simulink model "ADMIRE"  (R2021b)
settings: Solver=ode4  StartTime=0.0  StopTime=100  FixedStep=1e-2  RelTol=1e-3
undefined symbols (not defined in the file or in its folder): admireDB, Earth, WGS84
libraries: simulink_extras x112, simulink x27, aerolibutil x4, dspsigops x4, aerolibfltsims x3, sharedtransform x2, aerolibtransform2 x2, aerolibatmos2 x1, matrix_library x1, sharedutil x1, aerolibanimutils x1, vrlib x1
(part 8 of 15)

== system ADMIRE/Aircraft/Aerodynamics/TangentialForceCoefficient/MachRegion3/Ctlg ==
  in_bus : Inport
  Abs : Abs
  Bus Selector : BusSelector  OutputSignals=AeroIn_Bus.angleOfAttack_deg,AeroIn_Bus.angleOfSideslip_deg,AeroIn_Bus.lg_bool
  CTLST_BETA_ALFA : Lookup_n-D  BreakpointsForDimension1=admireDB.aerodata_sym.CTLST.breakpoints.ALFA  BreakpointsForDimension2=admireDB.aerodata_sym.CTLST.breakpoints.BETA  BreakpointsForDimension3=[5, 7]  Table=admireDB.aerodata_sym.CTLST.newTable  ExtrapMethod=Clip  InternalRulePriority=Speed  RndMeth=Simplest  InputSameDT=on
      settings: InputPortMap=u0,u1
  Product : Product  Inputs=**
  Ctlg : Outport
  wires:
  Abs/1 -> CTLST_BETA_ALFA/2
  Bus Selector/3 -> Product/2  "<lg_bool>"
  CTLST_BETA_ALFA/1 -> Product/1
  in_bus/1 -> Bus Selector/1
  Bus Selector/2 -> Abs/1  "<angleOfSideslip_deg>"
  Bus Selector/1 -> CTLST_BETA_ALFA/1  "<angleOfAttack_deg>"
  Product/1 -> Ctlg/1

== system ADMIRE/Aircraft/Aerodynamics/TangentialForceCoefficient/MachRegion3/eoeff ==
  AeroIn_Bus : Inport
  Bus Selector : BusSelector  OutputSignals=mach_nd
  CTDEYODE_M : Lookup_n-D  NumberOfTableDimensions=1  BreakpointsForDimension1=admireDB.aerodata_sym.CTDEYODE.breakpoints.M  BreakpointsForDimension3=[5, 7]  Table=admireDB.aerodata_sym.CTDEYODE.newTable  ExtrapMethod=Clip  InternalRulePriority=Speed  RndMeth=Simplest  InputSameDT=on
  Constant : Constant
  Sum : Sum  Inputs=-+|
  eoeff : Outport
  eieff : Outport  Port=2
  wires:
  Sum/1 -> eieff/1
  CTDEYODE_M/1 -> eoeff/1, Sum/1
  Constant/1 -> Sum/2
  Bus Selector/1 -> CTDEYODE_M/1  "<mach_nd>"
  AeroIn_Bus/1 -> Bus Selector/1

== system ADMIRE/Aircraft/Aerodynamics/YawMomentCoefficient/MachRegion1/Cymbasic ==
  in_bus : Inport
  Bus Selector : BusSelector  OutputSignals=AeroIn_Bus.angleOfAttack_deg
  Cymbasic_ : Subsystem
  Cymbasic : Outport
  wires:
  Cymbasic_/1(Cymbasic) -> Cymbasic/1
  Bus Selector/1 -> Cymbasic_/1(angleOfAttack_deg)  "<angleOfAttack_deg>"
  in_bus/1 -> Bus Selector/1  "in_bus"

== system ADMIRE/Aircraft/Aerodynamics/YawMomentCoefficient/MachRegion1/Cymbcai ==
  in_bus : Inport
  Bus Selector : BusSelector  OutputSignals=AeroIn_Bus.cai,AeroIn_Bus.angleOfAttack_deg,AeroIn_Bus.angleOfSideslip_deg
  Cymbcai_ : Subsystem
  Cymbcai : Outport
  wires:
  Bus Selector/3 -> Cymbcai_/3(angleOfSideslip_deg)  "<angleOfSideslip_deg>"
  Bus Selector/2 -> Cymbcai_/2(angleOfAttack_deg)  "<angleOfAttack_deg>"
  Bus Selector/1 -> Cymbcai_/1(CAI)  "<cai>"
  in_bus/1 -> Bus Selector/1  "in_bus"
  Cymbcai_/1(Cymbcai) -> Cymbcai/1

== system ADMIRE/Aircraft/Aerodynamics/YawMomentCoefficient/MachRegion1/Cymbde ==
  in_bus : Inport
  Bus Selector : BusSelector  OutputSignals=AeroIn_Bus.angleOfAttack_deg,AeroIn_Bus.dEI,AeroIn_Bus.angleOfSideslip_deg,AeroIn_Bus.dEY,eieff,eoeff
  Cymbde_ : Subsystem
  Cymbde : Outport
  wires:
  Bus Selector/6 -> Cymbde_/6(eoeff)  "<eoeff>"
  Bus Selector/5 -> Cymbde_/5(eieff)  "<eieff>"
  Bus Selector/4 -> Cymbde_/4(dEY)  "<dEY>"
  Bus Selector/3 -> Cymbde_/3(angleOfSideslip_deg)  "<angleOfSideslip_deg>"
  Bus Selector/2 -> Cymbde_/2(dEI)  "<dEI>"
  Bus Selector/1 -> Cymbde_/1(angleOfAttack_deg)  "<angleOfAttack_deg>"
  Cymbde_/1(Cymbde) -> Cymbde/1
  in_bus/1 -> Bus Selector/1  "in_bus"

== system ADMIRE/Aircraft/Aerodynamics/YawMomentCoefficient/MachRegion1/Cymbdle ==
  in_bus : Inport
  Bus Selector : BusSelector  OutputSignals=AeroIn_Bus.angleOfAttack_deg,AeroIn_Bus.dEI,AeroIn_Bus.angleOfSideslip_deg,AeroIn_Bus.lef_deg,AeroIn_Bus.dEY,eieff,eoeff
  Cymbdle_ : Subsystem
  Cymbdle : Outport
  wires:
  Bus Selector/2 -> Cymbdle_/2(dEI)  "<dEI>"
  Bus Selector/1 -> Cymbdle_/1(angleOfAttack_deg)  "<angleOfAttack_deg>"
  Bus Selector/3 -> Cymbdle_/3(angleOfSideslip_deg)  "<angleOfSideslip_deg>"
  Bus Selector/4 -> Cymbdle_/4(dLE)  "<lef_deg>"
  Bus Selector/5 -> Cymbdle_/5(dEY)  "<dEY>"
  Bus Selector/6 -> Cymbdle_/6(eieff)  "<eieff>"
  Bus Selector/7 -> Cymbdle_/7(eoeff)  "<eoeff>"
  Cymbdle_/1(Cymbdle) -> Cymbdle/1
  in_bus/1 -> Bus Selector/1  "in_bus"

== system ADMIRE/Aircraft/Aerodynamics/YawMomentCoefficient/MachRegion1/Cymbdn ==
  in_bus : Inport
  Bus Selector : BusSelector  OutputSignals=AeroIn_Bus.angleOfAttack_deg,AeroIn_Bus.dN,AeroIn_Bus.angleOfSideslip_deg
  Cymbdn_ : Subsystem
  Cymbdn : Outport
  wires:
  Bus Selector/1 -> Cymbdn_/1(angleOfAttack_deg)  "<angleOfAttack_deg>"
  Bus Selector/3 -> Cymbdn_/3(angleOfSideslip_deg)  "<angleOfSideslip_deg>"
  Bus Selector/2 -> Cymbdn_/2(dN)  "<dN>"
  in_bus/1 -> Bus Selector/1  "in_bus"
  Cymbdn_/1(Cymbdn) -> Cymbdn/1

== system ADMIRE/Aircraft/Aerodynamics/YawMomentCoefficient/MachRegion1/Cymbeta ==
  in_bus : Inport
  Bus Selector : BusSelector  OutputSignals=AeroIn_Bus.angleOfSideslip_deg,AeroIn_Bus.angleOfAttack_deg,AeroIn_Bus.qacorr,AeroIn_Bus.mach_nd
  Cymbeta_ : Subsystem
  Cymbeta : Outport
  wires:
  Bus Selector/4 -> Cymbeta_/4(mach_nd)  "<mach_nd>"
  Bus Selector/3 -> Cymbeta_/3(qacorr)  "<qacorr>"
  Bus Selector/2 -> Cymbeta_/2(angleOfAttack_deg)  "<angleOfAttack_deg>"
  Bus Selector/1 -> Cymbeta_/1(angleOfSideslip_deg)  "<angleOfSideslip_deg>"
  in_bus/1 -> Bus Selector/1  "in_bus"
  Cymbeta_/1(Cymbeta) -> Cymbeta/1

== system ADMIRE/Aircraft/Aerodynamics/YawMomentCoefficient/MachRegion1/Cymbetad ==
  in_bus : Inport
  Bus Selector : BusSelector  OutputSignals=AeroIn_Bus.angleOfAttack_deg,AeroIn_Bus.betad
  Cymbetad_ : Subsystem
  Cymbetad : Outport
  wires:
  Bus Selector/1 -> Cymbetad_/1(angleOfAttack_deg)  "<angleOfAttack_deg>"
  Bus Selector/2 -> Cymbetad_/2(betad)  "<betad>"
  Cymbetad_/1(Cymbetad) -> Cymbetad/1
  in_bus/1 -> Bus Selector/1  "in_bus"

== system ADMIRE/Aircraft/Aerodynamics/YawMomentCoefficient/MachRegion1/Cymblg ==
  in_bus : Inport
  Bus Selector : BusSelector  OutputSignals=AeroIn_Bus.angleOfSideslip_deg,AeroIn_Bus.lg_bool,AeroIn_Bus.angleOfAttack_deg
  Cymblg_ : Subsystem
  Cymblg : Outport
  wires:
  Bus Selector/3 -> Cymblg_/3(angleOfAttack_deg)  "<angleOfAttack_deg>"
  Bus Selector/1 -> Cymblg_/1(angleOfSideslip_deg)  "<angleOfSideslip_deg>"
  Bus Selector/2 -> Cymblg_/2(dLG)  "<lg_bool>"
  Cymblg_/1(Cymblg) -> Cymblg/1
  in_bus/1 -> Bus Selector/1  "in_bus"

== system ADMIRE/Aircraft/Aerodynamics/YawMomentCoefficient/MachRegion1/Cymdai ==
  in_bus : Inport
  Bus Selector : BusSelector  OutputSignals=AeroIn_Bus.dAI,AeroIn_Bus.angleOfAttack_deg,AeroIn_Bus.dEI,eieff,AeroIn_Bus.qacorr,AeroIn_Bus.mach_nd
  Cymdai_ : Subsystem
  Cymdai : Outport
  wires:
  Bus Selector/1 -> Cymdai_/1(dAI)  "<dAI>"
  Bus Selector/2 -> Cymdai_/2(angleOfAttack_deg)  "<angleOfAttack_deg>"
  Bus Selector/3 -> Cymdai_/3(dEI)  "<dEI>"
  Bus Selector/4 -> Cymdai_/4(eieff)  "<eieff>"
  Bus Selector/5 -> Cymdai_/5(qacorr)  "<qacorr>"
  Bus Selector/6 -> Cymdai_/6(mach_nd)  "<mach_nd>"
  Cymdai_/1(Cymdai) -> Cymdai/1
  in_bus/1 -> Bus Selector/1  "in_bus"

== system ADMIRE/Aircraft/Aerodynamics/YawMomentCoefficient/MachRegion1/Cymdaib ==
  in_bus : Inport
  Bus Selector : BusSelector  OutputSignals=AeroIn_Bus.angleOfAttack_deg,AeroIn_Bus.dAI,AeroIn_Bus.angleOfSideslip_deg,eieff
  Cymdaib_ : Subsystem
  Cymdaib : Outport
  wires:
  Bus Selector/4 -> Cymdaib_/4(eieff)  "<eieff>"
  Bus Selector/3 -> Cymdaib_/3(angleOfSideslip_deg)  "<angleOfSideslip_deg>"
  Bus Selector/2 -> Cymdaib_/2(dAI)  "<dAI>"
  Bus Selector/1 -> Cymdaib_/1(angleOfAttack_deg)  "<angleOfAttack_deg>"
  Cymdaib_/1(Cymdaib) -> Cymdaib/1
  in_bus/1 -> Bus Selector/1  "in_bus"

== system ADMIRE/Aircraft/Aerodynamics/YawMomentCoefficient/MachRegion1/Cymday ==
  in_bus : Inport
  Bus Selector : BusSelector  OutputSignals=AeroIn_Bus.dAY,AeroIn_Bus.angleOfAttack_deg,AeroIn_Bus.dEY,eoeff,AeroIn_Bus.qacorr,AeroIn_Bus.mach_nd
  Cymday_ : Subsystem
  Cymday : Outport
  wires:
  Bus Selector/1 -> Cymday_/1(dAY)  "<dAY>"
  Bus Selector/2 -> Cymday_/2(angleOfAttack_deg)  "<angleOfAttack_deg>"
  Bus Selector/3 -> Cymday_/3(dEY)  "<dEY>"
  Bus Selector/4 -> Cymday_/4(eoeff)  "<eoeff>"
  Bus Selector/5 -> Cymday_/5(qacorr)  "<qacorr>"
  Bus Selector/6 -> Cymday_/6(mach_nd)  "<mach_nd>"
  in_bus/1 -> Bus Selector/1  "in_bus"
  Cymday_/1(Cymday) -> Cymday/1

== system ADMIRE/Aircraft/Aerodynamics/YawMomentCoefficient/MachRegion1/Cymdayb ==
  in_bus : Inport
  Bus Selector : BusSelector  OutputSignals=AeroIn_Bus.angleOfAttack_deg,AeroIn_Bus.dAY,AeroIn_Bus.angleOfSideslip_deg,eoeff
  Cymdayb_ : Subsystem
  Cymdayb : Outport
  wires:
  Bus Selector/4 -> Cymdayb_/4(eoeff)  "<eoeff>"
  Bus Selector/3 -> Cymdayb_/3(angleOfSideslip_deg)  "<angleOfSideslip_deg>"
  Bus Selector/2 -> Cymdayb_/2(dAY)  "<dAY>"
  Bus Selector/1 -> Cymdayb_/1(angleOfAttack_deg)  "<angleOfAttack_deg>"
  Cymdayb_/1(Cymdaib) -> Cymdayb/1
  in_bus/1 -> Bus Selector/1  "in_bus"

== system ADMIRE/Aircraft/Aerodynamics/YawMomentCoefficient/MachRegion1/Cymdna ==
  in_bus : Inport
  Bus Selector : BusSelector  OutputSignals=AeroIn_Bus.dNE,AeroIn_Bus.angleOfAttack_deg,AeroIn_Bus.dNA
  Cymdna_ : Subsystem
  Cymdna : Outport
  wires:
  Bus Selector/3 -> Cymdna_/3(dNA)  "<dNA>"
  Bus Selector/2 -> Cymdna_/2(angleOfAttack_deg)  "<angleOfAttack_deg>"
  Bus Selector/1 -> Cymdna_/1(dNE)  "<dNE>"
  in_bus/1 -> Bus Selector/1  "in_bus"
  Cymdna_/1(Cymdna) -> Cymdna/1

== system ADMIRE/Aircraft/Aerodynamics/YawMomentCoefficient/MachRegion1/Cymdr ==
  in_bus : Inport
  Bus Selector : BusSelector  OutputSignals=AeroIn_Bus.angleOfAttack_deg,AeroIn_Bus.rud_deg,AeroIn_Bus.angleOfSideslip_deg,AeroIn_Bus.qacorr,AeroIn_Bus.mach_nd
  Cymdr_ : Subsystem
  Cymdr : Outport
  wires:
  Bus Selector/5 -> Cymdr_/5(mach_nd)  "<mach_nd>"
  Bus Selector/4 -> Cymdr_/4(qacorr)  "<qacorr>"
  Bus Selector/3 -> Cymdr_/3(angleOfSideslip_deg)  "<angleOfSideslip_deg>"
  Bus Selector/2 -> Cymdr_/2(dR)  "<rud_deg>"
  Bus Selector/1 -> Cymdr_/1(angleOfAttack_deg)  "<angleOfAttack_deg>"
  in_bus/1 -> Bus Selector/1  "in_bus"
  Cymdr_/1(Cymdr) -> Cymdr/1

== system ADMIRE/Aircraft/Aerodynamics/YawMomentCoefficient/MachRegion1/Cymp ==
  in_bus : Inport
  Bus Selector : BusSelector  OutputSignals=AeroIn_Bus.dN,AeroIn_Bus.angleOfAttack_deg,AeroIn_Bus.qacorr,AeroIn_Bus.mach_nd,AeroIn_Bus.pc
  Cymp_ : Subsystem
  Cymp : Outport
  wires:
  Bus Selector/5 -> Cymp_/5(pc)  "<pc>"
  Bus Selector/4 -> Cymp_/4(mach_nd)  "<mach_nd>"
  Bus Selector/3 -> Cymp_/3(qacorr)  "<qacorr>"
  Bus Selector/2 -> Cymp_/2(angleOfAttack_deg)  "<angleOfAttack_deg>"
  Bus Selector/1 -> Cymp_/1(dN)  "<dN>"
  in_bus/1 -> Bus Selector/1  "in_bus"
  Cymp_/1(Cymp) -> Cymp/1

== system ADMIRE/Aircraft/Aerodynamics/YawMomentCoefficient/MachRegion1/Cympbeta ==
  in_bus : Inport
  Bus Selector : BusSelector  OutputSignals=AeroIn_Bus.angleOfSideslip_deg,AeroIn_Bus.angleOfAttack_deg,AeroIn_Bus.pc
  Cympbeta_ : Subsystem
  Cympbeta : Outport
  wires:
  Bus Selector/3 -> Cympbeta_/3(pc)  "<pc>"
  Bus Selector/2 -> Cympbeta_/2(angleOfAttack_deg)  "<angleOfAttack_deg>"
  Bus Selector/1 -> Cympbeta_/1(angleOfSideslip_deg)  "<angleOfSideslip_deg>"
  Cympbeta_/1(Cympbeta) -> Cympbeta/1
  in_bus/1 -> Bus Selector/1  "in_bus"

== system ADMIRE/Aircraft/Aerodynamics/YawMomentCoefficient/MachRegion1/Cymr ==
  in_bus : Inport
  Bus Selector : BusSelector  OutputSignals=AeroIn_Bus.dN,AeroIn_Bus.angleOfAttack_deg,AeroIn_Bus.rc,AeroIn_Bus.mach_nd,AeroIn_Bus.qacorr
  Cymr_ : Subsystem
  Cymr : Outport
  wires:
  Bus Selector/5 -> Cymr_/5(qacorr)  "<qacorr>"
  Bus Selector/4 -> Cymr_/4(mach_nd)  "<mach_nd>"
  Bus Selector/3 -> Cymr_/3(rc)  "<rc>"
  Bus Selector/2 -> Cymr_/2(angleOfAttack_deg)  "<angleOfAttack_deg>"
  Bus Selector/1 -> Cymr_/1(dN)  "<dN>"
  in_bus/1 -> Bus Selector/1  "in_bus"
  Cymr_/1(Cymr) -> Cymr/1

== system ADMIRE/Aircraft/Aerodynamics/YawMomentCoefficient/MachRegion1/Cymrbeta ==
  in_bus : Inport
  Bus Selector : BusSelector  OutputSignals=AeroIn_Bus.angleOfSideslip_deg,AeroIn_Bus.angleOfAttack_deg,AeroIn_Bus.rc
  Cymrbeta_ : Subsystem
  Cymrbeta : Outport
  wires:
  Bus Selector/3 -> Cymrbeta_/3(rc)  "<rc>"
  Bus Selector/2 -> Cymrbeta_/2(angleOfAttack_deg)  "<angleOfAttack_deg>"
  Bus Selector/1 -> Cymrbeta_/1(angleOfSideslip_deg)  "<angleOfSideslip_deg>"
  Cymrbeta_/1(Cymrbeta) -> Cymrbeta/1
  in_bus/1 -> Bus Selector/1  "in_bus"

== system ADMIRE/Aircraft/Aerodynamics/YawMomentCoefficient/MachRegion1/eoeff ==
  AeroIn_Bus : Inport
  Bus Selector : BusSelector  OutputSignals=mach_nd
  CYMDAYOD_M : Lookup_n-D  NumberOfTableDimensions=1  BreakpointsForDimension1=admireDB.aerodata_asym_ext.CYMDAYOD.breakpoints.M  BreakpointsForDimension3=[5, 7]  Table=admireDB.aerodata_asym_ext.CYMDAYOD.newTable  ExtrapMethod=Clip  InternalRulePriority=Speed  RndMeth=Simplest  InputSameDT=on
  Constant : Constant
  Sum : Sum  Inputs=-+|
  eoeff : Outport
  eieff : Outport  Port=2
  wires:
  Sum/1 -> eieff/1
  CYMDAYOD_M/1 -> eoeff/1, Sum/1
  Constant/1 -> Sum/2
  Bus Selector/1 -> CYMDAYOD_M/1  "<mach_nd>"
  AeroIn_Bus/1 -> Bus Selector/1

== system ADMIRE/Aircraft/Aerodynamics/YawMomentCoefficient/MachRegion2/Cymbasic ==
  in_bus : Inport
  Bus Selector : BusSelector  OutputSignals=AeroIn_Bus.angleOfAttack_deg,AeroIn_Bus.tflow
  Cymbasic_ : Subsystem
  Cymbasic : Outport
  wires:
  Bus Selector/2 -> Cymbasic_/2(tflow)  "<tflow>"
  Cymbasic_/1(Cymbasic) -> Cymbasic/1
  Bus Selector/1 -> Cymbasic_/1(angleOfAttack_deg)  "<angleOfAttack_deg>"
  in_bus/1 -> Bus Selector/1  "in_bus"

== system ADMIRE/Aircraft/Aerodynamics/YawMomentCoefficient/MachRegion2/Cymbcai ==
  in_bus : Inport
  Bus Selector : BusSelector  OutputSignals=AeroIn_Bus.cai,AeroIn_Bus.angleOfAttack_deg,AeroIn_Bus.angleOfSideslip_deg
  Cymbcai_ : Subsystem
  Cymbcai : Outport
  wires:
  Bus Selector/3 -> Cymbcai_/3(angleOfSideslip_deg)  "<angleOfSideslip_deg>"
  Bus Selector/2 -> Cymbcai_/2(angleOfAttack_deg)  "<angleOfAttack_deg>"
  Bus Selector/1 -> Cymbcai_/1(CAI)  "<cai>"
  in_bus/1 -> Bus Selector/1  "in_bus"
  Cymbcai_/1(Cymbcai) -> Cymbcai/1

== system ADMIRE/Aircraft/Aerodynamics/YawMomentCoefficient/MachRegion2/Cymbde ==
  in_bus : Inport
  Bus Selector : BusSelector  OutputSignals=AeroIn_Bus.angleOfAttack_deg,AeroIn_Bus.dEI,AeroIn_Bus.angleOfSideslip_deg,AeroIn_Bus.dEY,eieff,eoeff
  Cymbde_ : Subsystem
  Cymbde : Outport
  wires:
  Bus Selector/6 -> Cymbde_/6(eoeff)  "<eoeff>"
  Bus Selector/5 -> Cymbde_/5(eieff)  "<eieff>"
  Bus Selector/4 -> Cymbde_/4(dEY)  "<dEY>"
  Bus Selector/3 -> Cymbde_/3(angleOfSideslip_deg)  "<angleOfSideslip_deg>"
  Bus Selector/2 -> Cymbde_/2(dEI)  "<dEI>"
  Bus Selector/1 -> Cymbde_/1(angleOfAttack_deg)  "<angleOfAttack_deg>"
  Cymbde_/1(Cymbde) -> Cymbde/1
  in_bus/1 -> Bus Selector/1  "in_bus"

== system ADMIRE/Aircraft/Aerodynamics/YawMomentCoefficient/MachRegion2/Cymbdle ==
  in_bus : Inport
  Bus Selector : BusSelector  OutputSignals=AeroIn_Bus.angleOfAttack_deg,AeroIn_Bus.dEI,AeroIn_Bus.angleOfSideslip_deg,AeroIn_Bus.lef_deg,AeroIn_Bus.dEY,AeroIn_Bus.tflow,AeroIn_Bus.tfhigh
  Cymbdle_ : Subsystem
  Cymbdle : Outport
  wires:
  Bus Selector/2 -> Cymbdle_/2(dEI)  "<dEI>"
  Bus Selector/1 -> Cymbdle_/1(angleOfAttack_deg)  "<angleOfAttack_deg>"
  Bus Selector/3 -> Cymbdle_/3(angleOfSideslip_deg)  "<angleOfSideslip_deg>"
  Bus Selector/4 -> Cymbdle_/4(dLE)  "<lef_deg>"
  Bus Selector/5 -> Cymbdle_/5(dEY)  "<dEY>"
  Bus Selector/6 -> Cymbdle_/6(tflow)  "<tflow>"
  Bus Selector/7 -> Cymbdle_/7(tfhigh)  "<tfhigh>"
  Cymbdle_/1(Cymbdle) -> Cymbdle/1
  in_bus/1 -> Bus Selector/1  "in_bus"

== system ADMIRE/Aircraft/Aerodynamics/YawMomentCoefficient/MachRegion2/Cymbdn ==
  in_bus : Inport
  Bus Selector : BusSelector  OutputSignals=AeroIn_Bus.angleOfAttack_deg,AeroIn_Bus.dN,AeroIn_Bus.angleOfSideslip_deg
  Crmbdn_ : Subsystem
  Cymbdn : Outport
  wires:
  Bus Selector/1 -> Crmbdn_/1(angleOfAttack_deg)  "<angleOfAttack_deg>"
  Bus Selector/3 -> Crmbdn_/3(angleOfSideslip_deg)  "<angleOfSideslip_deg>"
  Bus Selector/2 -> Crmbdn_/2(dN)  "<dN>"
  in_bus/1 -> Bus Selector/1  "in_bus"
  Crmbdn_/1(Crmbdn) -> Cymbdn/1

== system ADMIRE/Aircraft/Aerodynamics/YawMomentCoefficient/MachRegion2/Cymbeta ==
  in_bus : Inport
  Bus Selector : BusSelector  OutputSignals=AeroIn_Bus.angleOfSideslip_deg,AeroIn_Bus.angleOfAttack_deg,AeroIn_Bus.qacorr,AeroIn_Bus.mach_nd,AeroIn_Bus.tflow,AeroIn_Bus.tfhigh
  Cymbeta_ : Subsystem
  Cymbeta : Outport
  wires:
  Bus Selector/1 -> Cymbeta_/1(angleOfSideslip_deg)  "<angleOfSideslip_deg>"
  Bus Selector/2 -> Cymbeta_/2(angleOfAttack_deg)  "<angleOfAttack_deg>"
  Bus Selector/3 -> Cymbeta_/3(qacorr)  "<qacorr>"
  Bus Selector/4 -> Cymbeta_/4(mach_nd)  "<mach_nd>"
  Bus Selector/5 -> Cymbeta_/5(tflow)  "<tflow>"
  Bus Selector/6 -> Cymbeta_/6(thigh)  "<tfhigh>"
  in_bus/1 -> Bus Selector/1  "in_bus"
  Cymbeta_/1(Cymbeta) -> Cymbeta/1

== system ADMIRE/Aircraft/Aerodynamics/YawMomentCoefficient/MachRegion2/Cymbetad ==
  in_bus : Inport
  Bus Selector : BusSelector  OutputSignals=AeroIn_Bus.angleOfAttack_deg,AeroIn_Bus.tflow,AeroIn_Bus.tfhigh,AeroIn_Bus.betad
  Cymbetad_ : Subsystem
  Cymbetad : Outport
  wires:
  Bus Selector/4 -> Cymbetad_/4(betad)  "<betad>"
  Bus Selector/3 -> Cymbetad_/3(tfhigh)  "<tfhigh>"
  Bus Selector/2 -> Cymbetad_/2(tflow)  "<tflow>"
  Bus Selector/1 -> Cymbetad_/1(angleOfAttack_deg)  "<angleOfAttack_deg>"
  Cymbetad_/1(Cymbetad) -> Cymbetad/1
  in_bus/1 -> Bus Selector/1  "in_bus"

== system ADMIRE/Aircraft/Aerodynamics/YawMomentCoefficient/MachRegion2/Cymblg ==
  in_bus : Inport
  Bus Selector : BusSelector  OutputSignals=AeroIn_Bus.lg_bool,AeroIn_Bus.angleOfAttack_deg,AeroIn_Bus.angleOfSideslip_deg
  Cymblg_ : Subsystem
  Cymblg : Outport
  wires:
  Bus Selector/1 -> Cymblg_/1(dLG)  "<lg_bool>"
  Bus Selector/2 -> Cymblg_/2(angleOfAttack_deg)  "<angleOfAttack_deg>"
  Bus Selector/3 -> Cymblg_/3(angleOfSideslip_deg)  "<angleOfSideslip_deg>"
  Cymblg_/1(Cymblg) -> Cymblg/1
  in_bus/1 -> Bus Selector/1  "in_bus"

== system ADMIRE/Aircraft/Aerodynamics/YawMomentCoefficient/MachRegion2/Cymdai ==
  in_bus : Inport
  Bus Selector : BusSelector  OutputSignals=AeroIn_Bus.dAI,AeroIn_Bus.angleOfAttack_deg,AeroIn_Bus.dEI,AeroIn_Bus.tflow,AeroIn_Bus.tfhigh,eieff,AeroIn_Bus.qacorr,AeroIn_Bus.mach_nd
  Cymdai_ : Subsystem
  Cymdai : Outport
  wires:
  Bus Selector/8 -> Cymdai_/8(mach_nd)  "<mach_nd>"
  Bus Selector/7 -> Cymdai_/7(qacorr)  "<qacorr>"
  Bus Selector/6 -> Cymdai_/6(eieff)  "<eieff>"
  Bus Selector/5 -> Cymdai_/5(tfhigh)  "<tfhigh>"
  Bus Selector/4 -> Cymdai_/4(tflow)  "<tflow>"
  Bus Selector/3 -> Cymdai_/3(dEI)  "<dEI>"
  Bus Selector/2 -> Cymdai_/2(angleOfAttack_deg)  "<angleOfAttack_deg>"
  Bus Selector/1 -> Cymdai_/1(dAI)  "<dAI>"
  Cymdai_/1(Cymdai) -> Cymdai/1
  in_bus/1 -> Bus Selector/1  "in_bus"

== system ADMIRE/Aircraft/Aerodynamics/YawMomentCoefficient/MachRegion2/Cymdaib ==
  in_bus : Inport
  Bus Selector : BusSelector  OutputSignals=AeroIn_Bus.angleOfAttack_deg,AeroIn_Bus.dAI,AeroIn_Bus.angleOfSideslip_deg,eieff,AeroIn_Bus.tflow
  Cymdaib_ : Subsystem
  Cymdaib : Outport
  wires:
  Bus Selector/1 -> Cymdaib_/1(angleOfAttack_deg)  "<angleOfAttack_deg>"
  Bus Selector/2 -> Cymdaib_/2(dAI)  "<dAI>"
  Bus Selector/3 -> Cymdaib_/3(angleOfSideslip_deg)  "<angleOfSideslip_deg>"
  Bus Selector/4 -> Cymdaib_/4(eieff)  "<eieff>"
  Bus Selector/5 -> Cymdaib_/5(tflow)  "<tflow>"
  Cymdaib_/1(Cymdaib) -> Cymdaib/1
  in_bus/1 -> Bus Selector/1  "in_bus"

== system ADMIRE/Aircraft/Aerodynamics/YawMomentCoefficient/MachRegion2/Cymday ==
  in_bus : Inport
  Bus Selector : BusSelector  OutputSignals=AeroIn_Bus.dAY,AeroIn_Bus.angleOfAttack_deg,AeroIn_Bus.dEY,eoeff,AeroIn_Bus.qacorr,AeroIn_Bus.mach_nd,AeroIn_Bus.tflow,AeroIn_Bus.tfhigh
  Cymday_ : Subsystem
  Cymday : Outport
  wires:
  Bus Selector/1 -> Cymday_/1(dAY)  "<dAY>"
  Bus Selector/2 -> Cymday_/2(angleOfAttack_deg)  "<angleOfAttack_deg>"
  Bus Selector/3 -> Cymday_/3(dEY)  "<dEY>"
  Bus Selector/4 -> Cymday_/4(eoeff)  "<eoeff>"
  Bus Selector/5 -> Cymday_/5(qacorr)  "<qacorr>"
  Bus Selector/6 -> Cymday_/6(mach_nd)  "<mach_nd>"
  Bus Selector/7 -> Cymday_/7(tflow)  "<tflow>"
  Bus Selector/8 -> Cymday_/8(tfhigh)  "<tfhigh>"
  in_bus/1 -> Bus Selector/1  "in_bus"
  Cymday_/1(Cymday) -> Cymday/1

== system ADMIRE/Aircraft/Aerodynamics/YawMomentCoefficient/MachRegion2/Cymdayb ==
  in_bus : Inport
  Bus Selector : BusSelector  OutputSignals=AeroIn_Bus.angleOfAttack_deg,AeroIn_Bus.dAY,AeroIn_Bus.angleOfSideslip_deg,eoeff,AeroIn_Bus.tflow
  Cymdayb_ : Subsystem
  Cymdayb : Outport
  wires:
  Bus Selector/1 -> Cymdayb_/1(angleOfAttack_deg)  "<angleOfAttack_deg>"
  Bus Selector/2 -> Cymdayb_/2(dAY)  "<dAY>"
  Bus Selector/3 -> Cymdayb_/3(angleOfSideslip_deg)  "<angleOfSideslip_deg>"
  Bus Selector/4 -> Cymdayb_/4(eoeff)  "<eoeff>"
  Bus Selector/5 -> Cymdayb_/5(tflow)  "<tflow>"
  Cymdayb_/1(Cymdayb) -> Cymdayb/1
  in_bus/1 -> Bus Selector/1  "in_bus"

== system ADMIRE/Aircraft/Aerodynamics/YawMomentCoefficient/MachRegion2/Cymdna ==
  in_bus : Inport
  Bus Selector : BusSelector  OutputSignals=AeroIn_Bus.dNE,AeroIn_Bus.angleOfAttack_deg,AeroIn_Bus.tflow,AeroIn_Bus.tfhigh,AeroIn_Bus.dNA
  Cymdna_ : Subsystem
  Cymdna : Outport
  wires:
  Bus Selector/2 -> Cymdna_/2(angleOfAttack_deg)  "<angleOfAttack_deg>"
  Bus Selector/1 -> Cymdna_/1(dNE)  "<dNE>"
  Bus Selector/3 -> Cymdna_/3(tflow)  "<tflow>"
  Bus Selector/4 -> Cymdna_/4(tfhigh)  "<tfhigh>"
  Bus Selector/5 -> Cymdna_/5(dNA)  "<dNA>"
  in_bus/1 -> Bus Selector/1  "in_bus"
  Cymdna_/1(Cymdna) -> Cymdna/1

== system ADMIRE/Aircraft/Aerodynamics/YawMomentCoefficient/MachRegion2/Cymdr ==
  in_bus : Inport
  Bus Selector : BusSelector  OutputSignals=AeroIn_Bus.angleOfAttack_deg,AeroIn_Bus.rud_deg,AeroIn_Bus.angleOfSideslip_deg,AeroIn_Bus.tflow,AeroIn_Bus.tfhigh,AeroIn_Bus.qacorr,AeroIn_Bus.mach_nd
  Cymdr_ : Subsystem
  Cymdr : Outport
  wires:
  Bus Selector/1 -> Cymdr_/1(angleOfAttack_deg)  "<angleOfAttack_deg>"
  Bus Selector/2 -> Cymdr_/2(dR)  "<rud_deg>"
  Bus Selector/3 -> Cymdr_/3(angleOfSideslip_deg)  "<angleOfSideslip_deg>"
  Bus Selector/4 -> Cymdr_/4(tfhigh)  "<tflow>"
  Bus Selector/5 -> Cymdr_/5(tflow)  "<tfhigh>"
  Bus Selector/6 -> Cymdr_/6(qacorr)  "<qacorr>"
  Bus Selector/7 -> Cymdr_/7(mach_nd)  "<mach_nd>"
  in_bus/1 -> Bus Selector/1  "in_bus"
  Cymdr_/1(Cymdr) -> Cymdr/1

== system ADMIRE/Aircraft/Aerodynamics/YawMomentCoefficient/MachRegion2/Cymp ==
  in_bus : Inport
  Bus Selector : BusSelector  OutputSignals=AeroIn_Bus.dN,AeroIn_Bus.angleOfAttack_deg,AeroIn_Bus.tflow,AeroIn_Bus.tfhigh,AeroIn_Bus.pc,AeroIn_Bus.qacorr,AeroIn_Bus.mach_nd
  Cymp_ : Subsystem
  Cymp : Outport
  wires:
  Bus Selector/1 -> Cymp_/1(dN)  "<dN>"
  Bus Selector/2 -> Cymp_/2(angleOfAttack_deg)  "<angleOfAttack_deg>"
  Bus Selector/7 -> Cymp_/7(mach_nd)  "<mach_nd>"
  Bus Selector/3 -> Cymp_/3(tflow)  "<tflow>"
  Bus Selector/6 -> Cymp_/6(qacorr)  "<qacorr>"
  Bus Selector/4 -> Cymp_/4(tfhigh)  "<tfhigh>"
  Bus Selector/5 -> Cymp_/5(pc)  "<pc>"
  in_bus/1 -> Bus Selector/1  "in_bus"
  Cymp_/1(Cymp) -> Cymp/1

== system ADMIRE/Aircraft/Aerodynamics/YawMomentCoefficient/MachRegion2/Cympbeta ==
  in_bus : Inport
  Bus Selector : BusSelector  OutputSignals=AeroIn_Bus.angleOfSideslip_deg,AeroIn_Bus.angleOfAttack_deg,AeroIn_Bus.pc,AeroIn_Bus.tflow
  Cympbeta_ : Subsystem
  Cympbeta : Outport
  wires:
  Bus Selector/1 -> Cympbeta_/1(angleOfSideslip_deg)  "<angleOfSideslip_deg>"
  Bus Selector/2 -> Cympbeta_/2(angleOfAttack_deg)  "<angleOfAttack_deg>"
  Bus Selector/3 -> Cympbeta_/3(pc)  "<pc>"
  Bus Selector/4 -> Cympbeta_/4(tflow)  "<tflow>"
  Cympbeta_/1(Cympbeta) -> Cympbeta/1
  in_bus/1 -> Bus Selector/1  "in_bus"

== system ADMIRE/Aircraft/Aerodynamics/YawMomentCoefficient/MachRegion2/Cymr ==
  in_bus : Inport
  Bus Selector : BusSelector  OutputSignals=AeroIn_Bus.dN,AeroIn_Bus.angleOfAttack_deg,AeroIn_Bus.tflow,AeroIn_Bus.tfhigh,AeroIn_Bus.rc,AeroIn_Bus.mach_nd,AeroIn_Bus.qacorr
  Cymr_ : Subsystem
  Cymr : Outport
  wires:
  Bus Selector/7 -> Cymr_/7(qacorr)  "<qacorr>"
  Bus Selector/6 -> Cymr_/6(mach_nd)  "<mach_nd>"
  Bus Selector/5 -> Cymr_/5(rc)  "<rc>"
  Bus Selector/4 -> Cymr_/4(tfhigh)  "<tfhigh>"
  Bus Selector/3 -> Cymr_/3(tflow)  "<tflow>"
  Bus Selector/2 -> Cymr_/2(angleOfAttack_deg)  "<angleOfAttack_deg>"
  Bus Selector/1 -> Cymr_/1(dN)  "<dN>"
  in_bus/1 -> Bus Selector/1  "in_bus"
  Cymr_/1(Cymr) -> Cymr/1

== system ADMIRE/Aircraft/Aerodynamics/YawMomentCoefficient/MachRegion2/Cymrbeta ==
  in_bus : Inport
  Bus Selector : BusSelector  OutputSignals=AeroIn_Bus.angleOfSideslip_deg,AeroIn_Bus.angleOfAttack_deg,AeroIn_Bus.rc,AeroIn_Bus.tflow
  Cymrbeta_ : Subsystem
  Cymrbeta : Outport
  wires:
  Bus Selector/1 -> Cymrbeta_/1(angleOfSideslip_deg)  "<angleOfSideslip_deg>"
  Bus Selector/2 -> Cymrbeta_/2(angleOfAttack_deg)  "<angleOfAttack_deg>"
  Bus Selector/3 -> Cymrbeta_/3(rc)  "<rc>"
  Bus Selector/4 -> Cymrbeta_/4(tflow)  "<tflow>"
  Cymrbeta_/1(Cymrbeta) -> Cymrbeta/1
  in_bus/1 -> Bus Selector/1  "in_bus"

== system ADMIRE/Aircraft/Aerodynamics/YawMomentCoefficient/MachRegion2/eoeff ==
  AeroIn_Bus : Inport
  Bus Selector : BusSelector  OutputSignals=mach_nd
  CYMDAYOD_M : Lookup_n-D  NumberOfTableDimensions=1  BreakpointsForDimension1=admireDB.aerodata_asym_ext.CYMDAYOD.breakpoints.M  BreakpointsForDimension3=[5, 7]  Table=admireDB.aerodata_asym_ext.CYMDAYOD.newTable  ExtrapMethod=Clip  InternalRulePriority=Speed  RndMeth=Simplest  InputSameDT=on
  Constant : Constant
  Sum : Sum  Inputs=-+|
  eoeff : Outport
  eieff : Outport  Port=2
  wires:
  Sum/1 -> eieff/1
  CYMDAYOD_M/1 -> eoeff/1, Sum/1
  Constant/1 -> Sum/2
  Bus Selector/1 -> CYMDAYOD_M/1  "<mach_nd>"
  AeroIn_Bus/1 -> Bus Selector/1

== system ADMIRE/Aircraft/Aerodynamics/YawMomentCoefficient/MachRegion3/Cymbasic ==
  Constant : Constant  Value=0
  Cymbasic : Outport
  wires:
  Constant/1 -> Cymbasic/1

== system ADMIRE/Aircraft/Aerodynamics/YawMomentCoefficient/MachRegion3/Cymbcai ==
  in_bus : Inport
  Bus Selector : BusSelector  OutputSignals=AeroIn_Bus.cai,AeroIn_Bus.angleOfAttack_deg,AeroIn_Bus.angleOfSideslip_deg
  Cymbcai_ : Subsystem
  Cymbcai : Outport
  wires:
  Bus Selector/3 -> Cymbcai_/3(angleOfSideslip_deg)  "<angleOfSideslip_deg>"
  Bus Selector/2 -> Cymbcai_/2(angleOfAttack_deg)  "<angleOfAttack_deg>"
  Bus Selector/1 -> Cymbcai_/1(CAI)  "<cai>"
  in_bus/1 -> Bus Selector/1  "in_bus"
  Cymbcai_/1(Cymbcai) -> Cymbcai/1

== system ADMIRE/Aircraft/Aerodynamics/YawMomentCoefficient/MachRegion3/Cymbde ==
  in_bus : Inport
  Bus Selector : BusSelector  OutputSignals=AeroIn_Bus.angleOfAttack_deg,AeroIn_Bus.dEI,AeroIn_Bus.angleOfSideslip_deg,AeroIn_Bus.dEY,eieff,eoeff,AeroIn_Bus.mach_nd
  Cymbde_ : Subsystem
  Cymbde : Outport
  wires:
  Bus Selector/7 -> Cymbde_/7(mach_nd)  "<mach_nd>"
  Bus Selector/6 -> Cymbde_/6(eoeff)  "<eoeff>"
  Bus Selector/5 -> Cymbde_/5(eieff)  "<eieff>"
  Bus Selector/4 -> Cymbde_/4(dEY)  "<dEY>"
  Bus Selector/3 -> Cymbde_/3(angleOfSideslip_deg)  "<angleOfSideslip_deg>"
  Bus Selector/2 -> Cymbde_/2(dEI)  "<dEI>"
  Bus Selector/1 -> Cymbde_/1(angleOfAttack_deg)  "<angleOfAttack_deg>"
  Cymbde_/1(Cymbde) -> Cymbde/1
  in_bus/1 -> Bus Selector/1  "in_bus"

== system ADMIRE/Aircraft/Aerodynamics/YawMomentCoefficient/MachRegion3/Cymbdle ==
  in_bus : Inport
  Bus Selector : BusSelector  OutputSignals=AeroIn_Bus.angleOfAttack_deg,AeroIn_Bus.dEI,AeroIn_Bus.mach_nd,AeroIn_Bus.dEY,eieff,eoeff,AeroIn_Bus.angleOfSideslip_deg,AeroIn_Bus.lef_deg
  Cymbdle_ : Subsystem
  Cymbdle : Outport
  wires:
  Bus Selector/8 -> Cymbdle_/8(dLE)  "<lef_deg>"
  Bus Selector/7 -> Cymbdle_/7(angleOfSideslip_deg)  "<angleOfSideslip_deg>"
  Bus Selector/6 -> Cymbdle_/6(eoeff)  "<eoeff>"
  Bus Selector/5 -> Cymbdle_/5(eieff)  "<eieff>"
  Bus Selector/4 -> Cymbdle_/4(dEY)  "<dEY>"
  Bus Selector/3 -> Cymbdle_/3(mach_nd)  "<mach_nd>"
  Bus Selector/2 -> Cymbdle_/2(dEI)  "<dEI>"
  Bus Selector/1 -> Cymbdle_/1(angleOfAttack_deg)  "<angleOfAttack_deg>"
  Cymbdle_/1(Cymbdle) -> Cymbdle/1
  in_bus/1 -> Bus Selector/1  "in_bus"

== system ADMIRE/Aircraft/Aerodynamics/YawMomentCoefficient/MachRegion3/Cymbdn ==
  in_bus : Inport
  Bus Selector : BusSelector  OutputSignals=AeroIn_Bus.angleOfAttack_deg,AeroIn_Bus.dN,AeroIn_Bus.angleOfSideslip_deg
  Cymbdn_ : Subsystem
  Cymbdn : Outport
  wires:
  Bus Selector/1 -> Cymbdn_/1(angleOfAttack_deg)  "<angleOfAttack_deg>"
  Bus Selector/3 -> Cymbdn_/3(angleOfSideslip_deg)  "<angleOfSideslip_deg>"
  Bus Selector/2 -> Cymbdn_/2(dN)  "<dN>"
  in_bus/1 -> Bus Selector/1  "in_bus"
  Cymbdn_/1(Cymbdn) -> Cymbdn/1

== system ADMIRE/Aircraft/Aerodynamics/YawMomentCoefficient/MachRegion3/Cymbeta ==
  in_bus : Inport
  Bus Selector : BusSelector  OutputSignals=AeroIn_Bus.angleOfSideslip_deg,AeroIn_Bus.angleOfAttack_deg,AeroIn_Bus.mach_nd,AeroIn_Bus.qacorr
  Cymbeta_ : Subsystem
  Cymbeta : Outport
  wires:
  Bus Selector/1 -> Cymbeta_/1(angleOfSideslip_deg)  "<angleOfSideslip_deg>"
  Bus Selector/2 -> Cymbeta_/2(angleOfAttack_deg)  "<angleOfAttack_deg>"
  Bus Selector/3 -> Cymbeta_/3(mach_nd)  "<mach_nd>"
  Bus Selector/4 -> Cymbeta_/4(qacorr)  "<qacorr>"
  in_bus/1 -> Bus Selector/1  "in_bus"
  Cymbeta_/1(Cymbeta) -> Cymbeta/1

== system ADMIRE/Aircraft/Aerodynamics/YawMomentCoefficient/MachRegion3/Cymbetad ==
  in_bus : Inport
  Bus Selector : BusSelector  OutputSignals=AeroIn_Bus.angleOfAttack_deg,AeroIn_Bus.mach_nd,AeroIn_Bus.betad
  Cymbetad_ : Subsystem
  Cymbetad : Outport
  wires:
  Bus Selector/3 -> Cymbetad_/3(betad)  "<betad>"
  Bus Selector/2 -> Cymbetad_/2(mach_nd)  "<mach_nd>"
  Bus Selector/1 -> Cymbetad_/1(angleOfAttack_deg)  "<angleOfAttack_deg>"
  Cymbetad_/1(Cymbetad) -> Cymbetad/1
  in_bus/1 -> Bus Selector/1  "in_bus"

== system ADMIRE/Aircraft/Aerodynamics/YawMomentCoefficient/MachRegion3/Cymblg ==
  in_bus : Inport
  Bus Selector : BusSelector  OutputSignals=AeroIn_Bus.angleOfSideslip_deg,AeroIn_Bus.lg_bool,AeroIn_Bus.angleOfAttack_deg
  Cymblg_ : Subsystem
  Cymblg : Outport
  wires:
  Bus Selector/3 -> Cymblg_/3(angleOfAttack_deg)  "<angleOfAttack_deg>"
  Bus Selector/1 -> Cymblg_/1(angleOfSideslip_deg)  "<angleOfSideslip_deg>"
  Bus Selector/2 -> Cymblg_/2(dLG)  "<lg_bool>"
  Cymblg_/1(Cymblg) -> Cymblg/1
  in_bus/1 -> Bus Selector/1  "in_bus"

== system ADMIRE/Aircraft/Aerodynamics/YawMomentCoefficient/MachRegion3/Cymdai ==
  in_bus : Inport
  Bus Selector : BusSelector  OutputSignals=AeroIn_Bus.angleOfAttack_deg,AeroIn_Bus.dAI,AeroIn_Bus.mach_nd,AeroIn_Bus.dEI,AeroIn_Bus.qacorr,eieff
  Cymdai_ : Subsystem
  Cymdai : Outport
  wires:
  Bus Selector/6 -> Cymdai_/6(eieff)  "<eieff>"
  Bus Selector/5 -> Cymdai_/5(qacorr)  "<qacorr>"
  Bus Selector/4 -> Cymdai_/4(dEI)  "<dEI>"
  Bus Selector/3 -> Cymdai_/3(mach_nd)  "<mach_nd>"
  Bus Selector/2 -> Cymdai_/2(dAI)  "<dAI>"
  Bus Selector/1 -> Cymdai_/1(angleOfAttack_deg)  "<angleOfAttack_deg>"
  Cymdai_/1(Cymdai) -> Cymdai/1
  in_bus/1 -> Bus Selector/1  "in_bus"

== system ADMIRE/Aircraft/Aerodynamics/YawMomentCoefficient/MachRegion3/Cymdaib ==
  Cymdaib_ : Constant  Value=0
  Cymdaib : Outport
  wires:
  Cymdaib_/1 -> Cymdaib/1

== system ADMIRE/Aircraft/Aerodynamics/YawMomentCoefficient/MachRegion3/Cymday ==
  in_bus : Inport
  Bus Selector : BusSelector  OutputSignals=AeroIn_Bus.angleOfAttack_deg,AeroIn_Bus.dAY,AeroIn_Bus.mach_nd,AeroIn_Bus.dEY,eoeff,AeroIn_Bus.qacorr
  Cymday_ : Subsystem
  Cymday : Outport
  wires:
  Bus Selector/6 -> Cymday_/6(qacorr)  "<qacorr>"
  Bus Selector/5 -> Cymday_/5(eoef)  "<eoeff>"
  Bus Selector/1 -> Cymday_/1(angleOfAttack_deg)  "<angleOfAttack_deg>"
  Bus Selector/4 -> Cymday_/4(dEY)  "<dEY>"
  Bus Selector/2 -> Cymday_/2(dAY)  "<dAY>"
  Bus Selector/3 -> Cymday_/3(mach_nd)  "<mach_nd>"
  in_bus/1 -> Bus Selector/1  "in_bus"
  Cymday_/1(Cymday) -> Cymday/1

== system ADMIRE/Aircraft/Aerodynamics/YawMomentCoefficient/MachRegion3/Cymdayb ==
  Cymdayb_ : Constant  Value=0
  Cymdayb : Outport
  wires:
  Cymdayb_/1 -> Cymdayb/1

== system ADMIRE/Aircraft/Aerodynamics/YawMomentCoefficient/MachRegion3/Cymdna ==
  in_bus : Inport
  Bus Selector : BusSelector  OutputSignals=AeroIn_Bus.angleOfAttack_deg,AeroIn_Bus.mach_nd,AeroIn_Bus.dNA
  Cymdna_ : Subsystem
  Cymdna : Outport
  wires:
  Bus Selector/1 -> Cymdna_/1(angleOfAttack_deg)  "<angleOfAttack_deg>"
  Bus Selector/2 -> Cymdna_/2(mach_nd)  "<mach_nd>"
  Bus Selector/3 -> Cymdna_/3(dNA)  "<dNA>"
  in_bus/1 -> Bus Selector/1  "in_bus"
  Cymdna_/1(Cymdna) -> Cymdna/1

== system ADMIRE/Aircraft/Aerodynamics/YawMomentCoefficient/MachRegion3/Cymdr ==
  in_bus : Inport
  Bus Selector : BusSelector  OutputSignals=AeroIn_Bus.angleOfAttack_deg,AeroIn_Bus.mach_nd,AeroIn_Bus.rud_deg,AeroIn_Bus.qacorr
  Cymdr_ : Subsystem
  Cymdr : Outport
  wires:
  Bus Selector/1 -> Cymdr_/1(angleOfAttack_deg)  "<angleOfAttack_deg>"
  Bus Selector/2 -> Cymdr_/2(mach_nd)  "<mach_nd>"
  Bus Selector/3 -> Cymdr_/3(dR)  "<rud_deg>"
  Bus Selector/4 -> Cymdr_/4(qacorr)  "<qacorr>"
  in_bus/1 -> Bus Selector/1  "in_bus"
  Cymdr_/1(Cymdr) -> Cymdr/1

== system ADMIRE/Aircraft/Aerodynamics/YawMomentCoefficient/MachRegion3/Cymp ==
  in_bus : Inport
  Bus Selector : BusSelector  OutputSignals=AeroIn_Bus.angleOfAttack_deg,AeroIn_Bus.mach_nd,AeroIn_Bus.qacorr,AeroIn_Bus.pc
  Cymp_ : Subsystem
  Cymp : Outport
  wires:
  Bus Selector/1 -> Cymp_/1(angleOfAttack_deg)  "<angleOfAttack_deg>"
  Bus Selector/2 -> Cymp_/2(mach_nd)  "<mach_nd>"
  Bus Selector/3 -> Cymp_/3(qacorr)  "<qacorr>"
  Bus Selector/4 -> Cymp_/4(pc)  "<pc>"
  in_bus/1 -> Bus Selector/1  "in_bus"
  Cymp_/1(Cymp) -> Cymp/1

== system ADMIRE/Aircraft/Aerodynamics/YawMomentCoefficient/MachRegion3/Cympbeta ==
  Cympbeta_ : Constant  Value=0
  Cympbeta : Outport
  wires:
  Cympbeta_/1 -> Cympbeta/1

== system ADMIRE/Aircraft/Aerodynamics/YawMomentCoefficient/MachRegion3/Cymr ==
  in_bus : Inport
  Bus Selector : BusSelector  OutputSignals=AeroIn_Bus.mach_nd,AeroIn_Bus.angleOfAttack_deg,AeroIn_Bus.dN,AeroIn_Bus.qacorr,AeroIn_Bus.rc
  Cymr_ : Subsystem
  Cymr : Outport
  wires:
  Bus Selector/1 -> Cymr_/1(mach_nd)  "<mach_nd>"
  Bus Selector/2 -> Cymr_/2(angleOfAttack_deg)  "<angleOfAttack_deg>"
  Bus Selector/3 -> Cymr_/3(dN)  "<dN>"
  Bus Selector/4 -> Cymr_/4(qacorr)  "<qacorr>"
  Bus Selector/5 -> Cymr_/5(rc)  "<rc>"
  in_bus/1 -> Bus Selector/1  "in_bus"
  Cymr_/1(Cymr) -> Cymr/1

== system ADMIRE/Aircraft/Aerodynamics/YawMomentCoefficient/MachRegion3/Cymrbeta ==
  Cymrbeta_ : Constant  Value=0
  Cymrbeta : Outport
  wires:
  Cymrbeta_/1 -> Cymrbeta/1

== system ADMIRE/Aircraft/Aerodynamics/YawMomentCoefficient/MachRegion3/eoeff ==
  AeroIn_Bus : Inport
  Bus Selector : BusSelector  OutputSignals=mach_nd
  CYMDAYOD_M : Lookup_n-D  NumberOfTableDimensions=1  BreakpointsForDimension1=admireDB.aerodata_asym_ext.CYMDAYOD.breakpoints.M  BreakpointsForDimension3=[5, 7]  Table=admireDB.aerodata_asym_ext.CYMDAYOD.newTable  ExtrapMethod=Clip  InternalRulePriority=Speed  RndMeth=Simplest  InputSameDT=on
  Constant : Constant
  Sum : Sum  Inputs=-+|
  eoeff : Outport
  eieff : Outport  Port=2
  wires:
  Sum/1 -> eieff/1
  CYMDAYOD_M/1 -> eoeff/1, Sum/1
  Constant/1 -> Sum/2
  Bus Selector/1 -> CYMDAYOD_M/1  "<mach_nd>"
  AeroIn_Bus/1 -> Bus Selector/1

== system ADMIRE/Aircraft/Aerodynamics/YawMomentCoefficient/MachRegion4/Cymbasic ==
  Constant : Constant  Value=0
  Cymbasic : Outport
  wires:
  Constant/1 -> Cymbasic/1

== system ADMIRE/Aircraft/Aerodynamics/YawMomentCoefficient/MachRegion4/Cymbcai ==
  in_bus : Inport
  Bus Selector : BusSelector  OutputSignals=AeroIn_Bus.cai,AeroIn_Bus.angleOfAttack_deg,AeroIn_Bus.angleOfSideslip_deg
  Cymbcai_ : Subsystem
  Cymbcai : Outport
  wires:
  Cymbcai_/1(Cymbcai) -> Cymbcai/1
  in_bus/1 -> Bus Selector/1  "in_bus"
  Bus Selector/1 -> Cymbcai_/1(CAI)  "<cai>"
  Bus Selector/2 -> Cymbcai_/2(angleOfAttack_deg)  "<angleOfAttack_deg>"
  Bus Selector/3 -> Cymbcai_/3(angleOfSideslip_deg)  "<angleOfSideslip_deg>"

== system ADMIRE/Aircraft/Aerodynamics/YawMomentCoefficient/MachRegion4/Cymbde ==
  in_bus : Inport
  Bus Selector : BusSelector  OutputSignals=AeroIn_Bus.angleOfAttack_deg,AeroIn_Bus.dEI,AeroIn_Bus.angleOfSideslip_deg,AeroIn_Bus.dEY,eieff,eoeff,AeroIn_Bus.mach_nd
  Cymbde_ : Subsystem
  Cymbde : Outport
  wires:
  in_bus/1 -> Bus Selector/1  "in_bus"
  Cymbde_/1(Cymbde) -> Cymbde/1
  Bus Selector/1 -> Cymbde_/1(angleOfAttack_deg)  "<angleOfAttack_deg>"
  Bus Selector/2 -> Cymbde_/2(dEI)  "<dEI>"
  Bus Selector/3 -> Cymbde_/3(angleOfSideslip_deg)  "<angleOfSideslip_deg>"
  Bus Selector/4 -> Cymbde_/4(dEY)  "<dEY>"
  Bus Selector/5 -> Cymbde_/5(eieff)  "<eieff>"
  Bus Selector/6 -> Cymbde_/6(eoeff)  "<eoeff>"
  Bus Selector/7 -> Cymbde_/7(mach_nd)  "<mach_nd>"

== system ADMIRE/Aircraft/Aerodynamics/YawMomentCoefficient/MachRegion4/Cymbdle ==
  in_bus : Inport
  Bus Selector : BusSelector  OutputSignals=AeroIn_Bus.angleOfAttack_deg,AeroIn_Bus.dEI,AeroIn_Bus.mach_nd,AeroIn_Bus.dEY,eieff,eoeff,AeroIn_Bus.angleOfSideslip_deg,AeroIn_Bus.lef_deg
  Cymbdle_ : Subsystem
  Cymbdle : Outport
  wires:
  in_bus/1 -> Bus Selector/1  "in_bus"
  Cymbdle_/1(Cymbdle) -> Cymbdle/1
  Bus Selector/1 -> Cymbdle_/1(angleOfAttack_deg)  "<angleOfAttack_deg>"
  Bus Selector/2 -> Cymbdle_/2(dEI)  "<dEI>"
  Bus Selector/3 -> Cymbdle_/3(mach_nd)  "<mach_nd>"
  Bus Selector/4 -> Cymbdle_/4(dEY)  "<dEY>"
  Bus Selector/5 -> Cymbdle_/5(eieff)  "<eieff>"
  Bus Selector/6 -> Cymbdle_/6(eoeff)  "<eoeff>"
  Bus Selector/7 -> Cymbdle_/7(angleOfSideslip_deg)  "<angleOfSideslip_deg>"
  Bus Selector/8 -> Cymbdle_/8(dLE)  "<lef_deg>"

== system ADMIRE/Aircraft/Aerodynamics/YawMomentCoefficient/MachRegion4/Cymbdn ==
  in_bus : Inport
  Bus Selector : BusSelector  OutputSignals=AeroIn_Bus.angleOfAttack_deg,AeroIn_Bus.dN,AeroIn_Bus.angleOfSideslip_deg
  Cymbdn_ : Subsystem
  Cymbdn : Outport
  wires:
  Cymbdn_/1(Cymbdn) -> Cymbdn/1
  in_bus/1 -> Bus Selector/1  "in_bus"
  Bus Selector/2 -> Cymbdn_/2(dN)  "<dN>"
  Bus Selector/3 -> Cymbdn_/3(angleOfSideslip_deg)  "<angleOfSideslip_deg>"
  Bus Selector/1 -> Cymbdn_/1(angleOfAttack_deg)  "<angleOfAttack_deg>"

== system ADMIRE/Aircraft/Aerodynamics/YawMomentCoefficient/MachRegion4/Cymbeta ==
  in_bus : Inport
  Bus Selector : BusSelector  OutputSignals=AeroIn_Bus.angleOfSideslip_deg,AeroIn_Bus.angleOfAttack_deg,AeroIn_Bus.mach_nd,AeroIn_Bus.qacorr
  Cymbeta_ : Subsystem
  Cymbeta : Outport
  wires:
  Cymbeta_/1(Cymbeta) -> Cymbeta/1
  in_bus/1 -> Bus Selector/1  "in_bus"
  Bus Selector/4 -> Cymbeta_/4(qacorr)  "<qacorr>"
  Bus Selector/3 -> Cymbeta_/3(mach_nd)  "<mach_nd>"
  Bus Selector/2 -> Cymbeta_/2(angleOfAttack_deg)  "<angleOfAttack_deg>"
  Bus Selector/1 -> Cymbeta_/1(angleOfSideslip_deg)  "<angleOfSideslip_deg>"

== system ADMIRE/Aircraft/Aerodynamics/YawMomentCoefficient/MachRegion4/Cymbetad ==
  in_bus : Inport
  Bus Selector : BusSelector  OutputSignals=AeroIn_Bus.angleOfAttack_deg,AeroIn_Bus.mach_nd,AeroIn_Bus.betad
  Cymbetad_ : Subsystem
  Cymbetad : Outport
  wires:
  in_bus/1 -> Bus Selector/1  "in_bus"
  Cymbetad_/1(Cymbetad) -> Cymbetad/1
  Bus Selector/1 -> Cymbetad_/1(angleOfAttack_deg)  "<angleOfAttack_deg>"
  Bus Selector/2 -> Cymbetad_/2(mach_nd)  "<mach_nd>"
  Bus Selector/3 -> Cymbetad_/3(betad)  "<betad>"

== system ADMIRE/Aircraft/Aerodynamics/YawMomentCoefficient/MachRegion4/Cymblg ==
  in_bus : Inport
  Bus Selector : BusSelector  OutputSignals=AeroIn_Bus.angleOfSideslip_deg,AeroIn_Bus.lg_bool,AeroIn_Bus.angleOfAttack_deg
  Cymblg_ : Subsystem
  Cymblg : Outport
  wires:
  in_bus/1 -> Bus Selector/1  "in_bus"
  Cymblg_/1(Cymblg) -> Cymblg/1
  Bus Selector/2 -> Cymblg_/2(dLG)  "<lg_bool>"
  Bus Selector/1 -> Cymblg_/1(angleOfSideslip_deg)  "<angleOfSideslip_deg>"
  Bus Selector/3 -> Cymblg_/3(angleOfAttack_deg)  "<angleOfAttack_deg>"

== system ADMIRE/Aircraft/Aerodynamics/YawMomentCoefficient/MachRegion4/Cymdai ==
  in_bus : Inport
  Bus Selector : BusSelector  OutputSignals=AeroIn_Bus.dAI,AeroIn_Bus.angleOfAttack_deg,AeroIn_Bus.dEI,AeroIn_Bus.mach_nd,eieff,AeroIn_Bus.qacorr
  Cymdai_ : Subsystem
  Cymdai : Outport
  wires:
  Bus Selector/1 -> Cymdai_/1(dAI)  "<dAI>"
  Bus Selector/2 -> Cymdai_/2(angleOfAttack_deg)  "<angleOfAttack_deg>"
  Bus Selector/3 -> Cymdai_/3(dEI)  "<dEI>"
  Bus Selector/4 -> Cymdai_/4(mach_nd)  "<mach_nd>"
  Bus Selector/5 -> Cymdai_/5(eieff)  "<eieff>"
  Bus Selector/6 -> Cymdai_/6(qacorr)  "<qacorr>"
  in_bus/1 -> Bus Selector/1  "in_bus"
  Cymdai_/1(Cymdai) -> Cymdai/1

== system ADMIRE/Aircraft/Aerodynamics/YawMomentCoefficient/MachRegion4/Cymdaib ==
  Cymdaib_ : Constant  Value=0
  Cymdaib : Outport
  wires:
  Cymdaib_/1 -> Cymdaib/1

== system ADMIRE/Aircraft/Aerodynamics/YawMomentCoefficient/MachRegion4/Cymday ==
  in_bus : Inport
  Bus Selector : BusSelector  OutputSignals=AeroIn_Bus.angleOfAttack_deg,AeroIn_Bus.dEY,AeroIn_Bus.mach_nd,AeroIn_Bus.qacorr,eoeff,AeroIn_Bus.dAY
  Cymday_ : Subsystem
  Cymday : Outport
  wires:
  Bus Selector/6 -> Cymday_/6(dAY)  "<dAY>"
  Bus Selector/5 -> Cymday_/5(eoeff)  "<eoeff>"
  Bus Selector/4 -> Cymday_/4(qacorr)  "<qacorr>"
  Bus Selector/3 -> Cymday_/3(mach_nd)  "<mach_nd>"
  Bus Selector/2 -> Cymday_/2(dEY)  "<dEY>"
  Bus Selector/1 -> Cymday_/1(angleOfAttack_deg)  "<angleOfAttack_deg>"
  Cymday_/1(Cymday) -> Cymday/1
  in_bus/1 -> Bus Selector/1  "in_bus"

== system ADMIRE/Aircraft/Aerodynamics/YawMomentCoefficient/MachRegion4/Cymdayb ==
  Cymdayb_ : Constant  Value=0
  Cymdayb : Outport
  wires:
  Cymdayb_/1 -> Cymdayb/1

== system ADMIRE/Aircraft/Aerodynamics/YawMomentCoefficient/MachRegion4/Cymdna ==
  in_bus : Inport
  Bus Selector : BusSelector  OutputSignals=AeroIn_Bus.angleOfAttack_deg,AeroIn_Bus.mach_nd,AeroIn_Bus.dNA
  Cymdna_ : Subsystem
  Cymdna : Outport
  wires:
  Cymdna_/1(Cymdna) -> Cymdna/1
  in_bus/1 -> Bus Selector/1  "in_bus"
  Bus Selector/3 -> Cymdna_/3(dNA)  "<dNA>"
  Bus Selector/2 -> Cymdna_/2(mach_nd)  "<mach_nd>"
  Bus Selector/1 -> Cymdna_/1(angleOfAttack_deg)  "<angleOfAttack_deg>"

== system ADMIRE/Aircraft/Aerodynamics/YawMomentCoefficient/MachRegion4/Cymdr ==
  in_bus : Inport
  Bus Selector : BusSelector  OutputSignals=AeroIn_Bus.angleOfAttack_deg,AeroIn_Bus.mach_nd,AeroIn_Bus.rud_deg,AeroIn_Bus.qacorr
  Cymdr_ : Subsystem
  Cymdr : Outport
  wires:
  Cymdr_/1(Cymdr) -> Cymdr/1
  in_bus/1 -> Bus Selector/1  "in_bus"
  Bus Selector/4 -> Cymdr_/4(qacorr)  "<qacorr>"
  Bus Selector/3 -> Cymdr_/3(dR)  "<rud_deg>"
  Bus Selector/2 -> Cymdr_/2(mach_nd)  "<mach_nd>"
  Bus Selector/1 -> Cymdr_/1(angleOfAttack_deg)  "<angleOfAttack_deg>"

== system ADMIRE/Aircraft/Aerodynamics/YawMomentCoefficient/MachRegion4/Cymp ==
  in_bus : Inport
  Bus Selector : BusSelector  OutputSignals=AeroIn_Bus.angleOfAttack_deg,AeroIn_Bus.mach_nd,AeroIn_Bus.qacorr,AeroIn_Bus.pc
  Cymp_ : Subsystem
  Cymp : Outport
  wires:
  Cymp_/1(Cymp) -> Cymp/1
  in_bus/1 -> Bus Selector/1  "in_bus"
  Bus Selector/4 -> Cymp_/4(pc)  "<pc>"
  Bus Selector/3 -> Cymp_/3(qacorr)  "<qacorr>"
  Bus Selector/2 -> Cymp_/2(mach_nd)  "<mach_nd>"
  Bus Selector/1 -> Cymp_/1(angleOfAttack_deg)  "<angleOfAttack_deg>"

== system ADMIRE/Aircraft/Aerodynamics/YawMomentCoefficient/MachRegion4/Cympbeta ==
  Cympbeta_ : Constant  Value=0
  Cympbeta : Outport
  wires:
  Cympbeta_/1 -> Cympbeta/1

== system ADMIRE/Aircraft/Aerodynamics/YawMomentCoefficient/MachRegion4/Cymr ==
  in_bus : Inport
  Bus Selector : BusSelector  OutputSignals=AeroIn_Bus.mach_nd,AeroIn_Bus.angleOfAttack_deg,AeroIn_Bus.dN,AeroIn_Bus.qacorr,AeroIn_Bus.rc
  Cymr_ : Subsystem
  Cymr : Outport
  wires:
  Cymr_/1(Cymr) -> Cymr/1
  in_bus/1 -> Bus Selector/1  "in_bus"
  Bus Selector/5 -> Cymr_/5(rc)  "<rc>"
  Bus Selector/4 -> Cymr_/4(qacorr)  "<qacorr>"
  Bus Selector/3 -> Cymr_/3(dN)  "<dN>"
  Bus Selector/2 -> Cymr_/2(angleOfAttack_deg)  "<angleOfAttack_deg>"
  Bus Selector/1 -> Cymr_/1(mach_nd)  "<mach_nd>"

== system ADMIRE/Aircraft/Aerodynamics/YawMomentCoefficient/MachRegion4/Cymrbeta ==
  Cymrbeta_ : Constant  Value=0
  Cymrbeta : Outport
  wires:
  Cymrbeta_/1 -> Cymrbeta/1

== system ADMIRE/Aircraft/Aerodynamics/YawMomentCoefficient/MachRegion4/eoeff ==
  AeroIn_Bus : Inport
  Bus Selector : BusSelector  OutputSignals=mach_nd
  CYMDAYOD_M : Lookup_n-D  NumberOfTableDimensions=1  BreakpointsForDimension1=admireDB.aerodata_asym_ext.CYMDAYOD.breakpoints.M  BreakpointsForDimension3=[5, 7]  Table=admireDB.aerodata_asym_ext.CYMDAYOD.newTable  ExtrapMethod=Clip  InternalRulePriority=Speed  RndMeth=Simplest  InputSameDT=on
  Constant : Constant
  Sum : Sum  Inputs=-+|
  eoeff : Outport
  eieff : Outport  Port=2
  wires:
  AeroIn_Bus/1 -> Bus Selector/1
  Bus Selector/1 -> CYMDAYOD_M/1  "<mach_nd>"
  Constant/1 -> Sum/2
  CYMDAYOD_M/1 -> Sum/1, eoeff/1
  Sum/1 -> eieff/1

== system ADMIRE/Aircraft/ControlSurfaces/Actuator/FirstOrder/canardL ==
  actIn : Inport
  Gain : Gain  Gain=20
  Saturation : Saturate  UpperLimit=60  LowerLimit=-60
  Saturation1 : Saturate  UpperLimit=25  LowerLimit=-25
  Sum : Sum  Inputs=|+-
  canardL_deg : Integrator
  actOut : Outport
  wires:
  actIn/1 -> Saturation1/1
  Sum/1 -> Gain/1
  Gain/1 -> Saturation/1
  Saturation/1 -> canardL_deg/1
  canardL_deg/1 -> Sum/2, actOut/1
  Saturation1/1 -> Sum/1

== system ADMIRE/Aircraft/ControlSurfaces/Actuator/FirstOrder/inElevonL ==
  actIn : Inport
  Gain : Gain  Gain=20
  Saturation : Saturate  UpperLimit=60  LowerLimit=-60
  Saturation1 : Saturate  UpperLimit=25  LowerLimit=-25
  Sum : Sum  Inputs=|+-
  inElevonL_deg : Integrator
  actOut : Outport
  wires:
  actIn/1 -> Saturation1/1
  Sum/1 -> Gain/1
  Gain/1 -> Saturation/1
  Saturation/1 -> inElevonL_deg/1
  inElevonL_deg/1 -> Sum/2, actOut/1
  Saturation1/1 -> Sum/1

== system ADMIRE/Aircraft/ControlSurfaces/Actuator/FirstOrder/inElevonR ==
  actIn : Inport
  Gain : Gain  Gain=20
  Saturation : Saturate  UpperLimit=60  LowerLimit=-60
  Saturation1 : Saturate  UpperLimit=25  LowerLimit=-25
  Sum : Sum  Inputs=|+-
  inElevonR_deg : Integrator
  actOut : Outport
  wires:
  Saturation1/1 -> Sum/1
  inElevonR_deg/1 -> actOut/1, Sum/2
  Saturation/1 -> inElevonR_deg/1
  Gain/1 -> Saturation/1
  Sum/1 -> Gain/1
  actIn/1 -> Saturation1/1

== system ADMIRE/Aircraft/ControlSurfaces/Actuator/FirstOrder/lef ==
  actIn : Inport
  Gain : Gain  Gain=20
  Saturation : Saturate  UpperLimit=60  LowerLimit=-60
  Saturation1 : Saturate  UpperLimit=25  LowerLimit=-25
  Sum : Sum  Inputs=|+-
  lef_deg : Integrator
  actOut : Outport
  wires:
  actIn/1 -> Saturation1/1
  Sum/1 -> Gain/1
  Gain/1 -> Saturation/1
  Saturation/1 -> lef_deg/1
  lef_deg/1 -> Sum/2, actOut/1
  Saturation1/1 -> Sum/1

== system ADMIRE/Aircraft/ControlSurfaces/Actuator/FirstOrder/outCanardR ==
  actIn : Inport
  Gain : Gain  Gain=20
  Saturation : Saturate  UpperLimit=60  LowerLimit=-60
  Saturation1 : Saturate  UpperLimit=25  LowerLimit=-25
  Sum : Sum  Inputs=|+-
  outCanardR_deg : Integrator
  actOut : Outport
  wires:
  Saturation1/1 -> Sum/1
  outCanardR_deg/1 -> actOut/1, Sum/2
  Saturation/1 -> outCanardR_deg/1
  Gain/1 -> Saturation/1
  Sum/1 -> Gain/1
  actIn/1 -> Saturation1/1

== system ADMIRE/Aircraft/ControlSurfaces/Actuator/FirstOrder/outElevonL ==
  actIn : Inport
  Gain : Gain  Gain=20
  Saturation : Saturate  UpperLimit=60  LowerLimit=-60
  Saturation1 : Saturate  UpperLimit=25  LowerLimit=-25
  Sum : Sum  Inputs=|+-
  outElevonL_deg : Integrator
  actOut : Outport
  wires:
  Saturation1/1 -> Sum/1
  outElevonL_deg/1 -> actOut/1, Sum/2
  Saturation/1 -> outElevonL_deg/1
  Gain/1 -> Saturation/1
  Sum/1 -> Gain/1
  actIn/1 -> Saturation1/1

== system ADMIRE/Aircraft/ControlSurfaces/Actuator/FirstOrder/outElevonR ==
  actIn : Inport
  Gain : Gain  Gain=20
  Saturation : Saturate  UpperLimit=60  LowerLimit=-60
  Saturation1 : Saturate  UpperLimit=25  LowerLimit=-25
  Sum : Sum  Inputs=|+-
  outElevonR_deg : Integrator
  actOut : Outport
  wires:
  actIn/1 -> Saturation1/1
  Sum/1 -> Gain/1
  Gain/1 -> Saturation/1
  Saturation/1 -> outElevonR_deg/1
  outElevonR_deg/1 -> Sum/2, actOut/1
  Saturation1/1 -> Sum/1

== system ADMIRE/Aircraft/ControlSurfaces/Actuator/FirstOrder/rudder ==
  actIn : Inport
  Gain : Gain  Gain=20
  Saturation : Saturate  UpperLimit=60  LowerLimit=-60
  Saturation1 : Saturate  UpperLimit=25  LowerLimit=-25
  Sum : Sum  Inputs=|+-
  rudder_deg : Integrator
  actOut : Outport
  wires:
  actIn/1 -> Saturation1/1
  Sum/1 -> Gain/1
  Gain/1 -> Saturation/1
  Saturation/1 -> rudder_deg/1
  rudder_deg/1 -> Sum/2, actOut/1
  Saturation1/1 -> Sum/1

== system ADMIRE/Aircraft/Aerodynamics/CentripetalForceCoefficient/MachRegion1/Ccbcai/Ccbcai_ ==
  CAI : Inport
  angleOfAttack_deg : Inport  Port=2
  angleOfSideslip_deg : Inport  Port=3
  CCBCAI_CAI_ALFA : Lookup_n-D  BreakpointsForDimension1=admireDB.aerodata_asym_ext.CCBCAI.breakpoints.ALFA  BreakpointsForDimension2=admireDB.aerodata_asym_ext.CCBCAI.breakpoints.CAI  BreakpointsForDimension3=[5, 7]  Table=admireDB.aerodata_asym_ext.CCBCAI.newTable  ExtrapMethod=Clip  InternalRulePriority=Speed  RndMeth=Simplest  InputSameDT=on
      settings: InputPortMap=u0,u1
  Degrees to Radians : simulink_extras/Transformations/Degrees to Radians
  Product : Product  Inputs=**
  Ccbcai : Outport
  wires:
  Degrees to Radians/1 -> Product/2
  angleOfSideslip_deg/1 -> Degrees to Radians/1
  Product/1 -> Ccbcai/1
  CCBCAI_CAI_ALFA/1 -> Product/1
  CAI/1 -> CCBCAI_CAI_ALFA/2
  angleOfAttack_deg/1 -> CCBCAI_CAI_ALFA/1
